simulink model "verify_Compression_Air_Water_Chiller_mdl"  (R2016b)
settings: Solver=ode45  StartTime=0  StopTime=1200  MaxStep=60  RelTol=1e-3  EnableMultiTasking=on
libraries: carnot x2
settings Model: Creator=drhf  LastModifiedBy=User
settings DataIOCC: SaveFormat=Array  SignalLoggingSaveFormat=ModelDataLogs
settings OptimizationCC: ExpressionDepthLimit=2147483647  LifeSpan=inf
settings DebuggingCC: UnderspecifiedInitializationDetection=Classic  MergeDetectMultiDrivingBlocksExec=none  SolverPrmCheckMsg=warning  FcnCallInpInsideContextMsg=warning  StateNameClashWarn=warning  SFUnexpectedBacktrackingDiag=warning  SFNoUnconditionalDefaultTransitionDiag=warning  SFExecutionAtInitializationDiag=none
settings HardwareCC: ProdBitPerPointer=32  ProdBitPerSizeT=32  ProdBitPerPtrDiffT=32  ProdLargestAtomicFloat=None  ProdIntDivRoundTo=Undefined  ProdEndianess=Unspecified  ProdWordSize=32  ProdHWDeviceType=32-bit Generic
settings ModelReferenceCC: PropagateSignalLabelsOutOfModel=off
settings GRTTargetCC: TargetLangStandard=C89/C90 (ANSI)  GeneratePreprocessorConditionals=Disable all  CombineOutputUpdateFcns=off  GRTInterface=on
settings ConfigComp: CovMetricSettings=dw  CovHtmlReporting=on  CovSaveCumulativeToWorkspaceVar=on  CovSaveSingleToWorkspaceVar=on  CovExternalEMLEnable=off

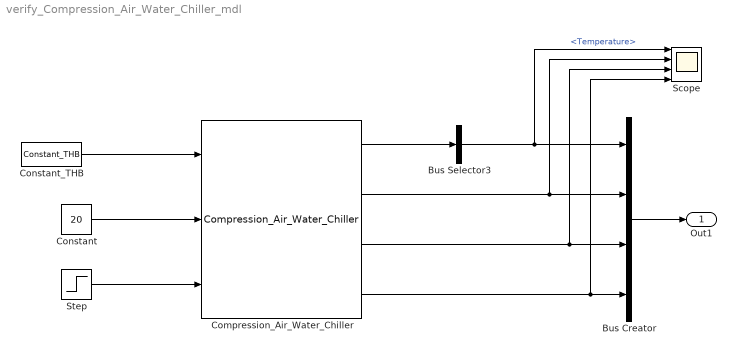
== system verify_Compression_Air_Water_Chiller_mdl ==
  Bus Creator : BusCreator  Inputs=4
  Bus Selector3 : BusSelector  OutputSignals=Temperature
  Compression_Air_Water_Chiller : carnot/Source/Chiller/Compression_Air_Water_Chiller  Q_Nom=15
  Constant : Constant  Value=20
  Constant_THB : carnot/Source/Simple/Constant_THB  t=40  mdot=1000/3600  p=2e5  mID=No Pressure Drop  fluid=Water  mix=0  mix2=0  mix3=0  dia=0.02  hgt=0
  Scope : Scope  NumInputPorts=4
  Step : Step  Time=0  SampleTime=0
  Out1 : Outport
  wires:
  Bus Creator/1 -> Out1/1
  Bus Selector3/1 -> Scope/1, Bus Creator/1  "<Temperature>"
  Constant_THB/1 -> Compression_Air_Water_Chiller/1
  Step/1 -> Compression_Air_Water_Chiller/3
  Compression_Air_Water_Chiller/2 -> Scope/2, Bus Creator/2
  Constant/1 -> Compression_Air_Water_Chiller/2
  Compression_Air_Water_Chiller/1 -> Bus Selector3/1
  Compression_Air_Water_Chiller/3 -> Scope/3, Bus Creator/3
  Compression_Air_Water_Chiller/4 -> Scope/4, Bus Creator/4
